simulink model "VariantSubsystem"  (R2015b)
settings: Solver=VariableStepAuto  StartTime=0.0  StopTime=10.0  RelTol=1e-3
undefined symbols (not defined in the file or in its folder): variant
settings Model: Creator=LUBO  LastModifiedBy=LUBO

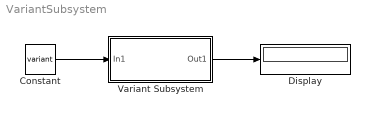
== system VariantSubsystem ==
  Constant : Constant  Value=variant
  Display : Display
  Variant Subsystem : Subsystem  Variant=on
  wires:
  Constant/1 -> Variant Subsystem/1(In1)
  Variant Subsystem/1(Out1) -> Display/1

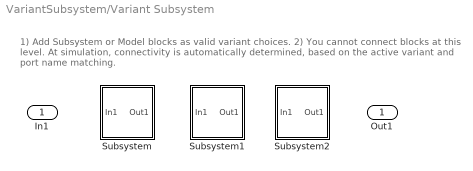
== system VariantSubsystem/Variant Subsystem ==
  note: 1) Add Subsystem or Model blocks as valid variant choices.
      | 2) You cannot connect blocks at this level. At simulation, connectivity is automatically
      | determined, based on the active variant and port name matching.
  In1 : Inport
  Subsystem : Subsystem  VariantControl=Variant1
  Subsystem1 : Subsystem  VariantControl=Variant2
  Subsystem2 : Subsystem  VariantControl=Variant3
  Out1 : Outport

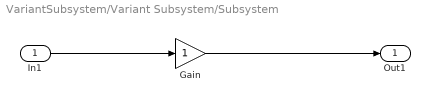
== system VariantSubsystem/Variant Subsystem/Subsystem ==
  In1 : Inport
  Gain : Gain
  Out1 : Outport
  wires:
  Gain/1 -> Out1/1
  In1/1 -> Gain/1

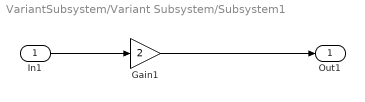
== system VariantSubsystem/Variant Subsystem/Subsystem1 ==
  In1 : Inport
  Gain1 : Gain  Gain=2
  Out1 : Outport
  wires:
  In1/1 -> Gain1/1
  Gain1/1 -> Out1/1

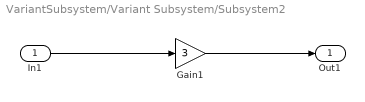
== system VariantSubsystem/Variant Subsystem/Subsystem2 ==
  In1 : Inport
  Gain1 : Gain  Gain=3
  Out1 : Outport
  wires:
  In1/1 -> Gain1/1
  Gain1/1 -> Out1/1
